simulink model "Modulation1"  (R2019b)
settings: Solver=VariableStepAuto  StartTime=0.0  StopTime=2  RelTol=1e-3
settings Model: Creator=Lenovo  LastModifiedBy=Lenovo

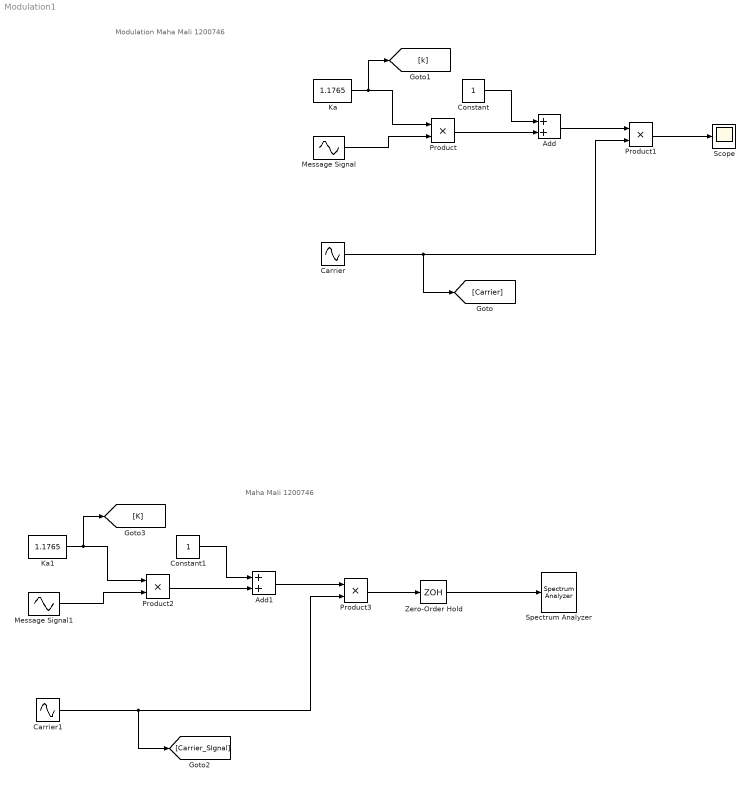
== system Modulation1 ==
  note: Maha Mali 1200746
  note: Modulation Maha Mali 1200746
  Add : Sum
  Add1 : Sum
  Carrier : Sin  Frequency=2*pi*15000  Phase=pi/2  SampleTime=0
  Carrier1 : Sin  Frequency=2*pi*15000  SampleTime=0
  Constant : Constant
  Constant1 : Constant
  Ka : Constant  Value=1.1765
  Ka1 : Constant  Value=1.1765
  Message Signal : Sin  Amplitude=0.85  Frequency=2*pi*1000  Phase=pi/2  SampleTime=0
  Message Signal1 : Sin  Amplitude=0.85  Frequency=2*pi*1000  SampleTime=0
  Product{,1..3} (4 alike) : Product
  Scope : Scope
  Spectrum Analyzer : SpectrumAnalyzer
  Zero-Order Hold : ZeroOrderHold  SampleTime=1/(10*15e3)
  wires:
  Product1/1 -> Scope/1
  Add/1 -> Product1/1
  Ka/1 -> [k], Product/1
  Product/1 -> Add/2
  Message Signal/1 -> Product/2
  Carrier/1 -> [Carrier], Product1/2
  Constant/1 -> Add/1
  Add1/1 -> Product3/1
  Ka1/1 -> [K], Product2/1
  Constant1/1 -> Add1/1
  Product2/1 -> Add1/2
  Message Signal1/1 -> Product2/2
  Carrier1/1 -> [Carrier_SIgnal], Product3/2
  Zero-Order Hold/1 -> Spectrum Analyzer/1
  Product3/1 -> Zero-Order Hold/1
